simulink model "adc1_sub_start"  (R2018b)
settings: Solver=ode45  StartTime=0.0  StopTime=10.0  RelTol=1e-3  EnableMultiTasking=on
libraries: dsparch4 x2
settings Model: Creator=bbhattac  LastModifiedBy=khung
settings DataIOCC: LimitDataPoints=on  SaveFormat=Array
settings OptimizationCC: ExpressionDepthLimit=2147483647  LifeSpan=inf
settings DebuggingCC: UnderspecifiedInitializationDetection=Classic  MergeDetectMultiDrivingBlocksExec=none  SolverPrmCheckMsg=warning  ParameterPrecisionLossMsg=none  StateNameClashWarn=warning  SFUnexpectedBacktrackingDiag=warning  SFNoUnconditionalDefaultTransitionDiag=warning  SFExecutionAtInitializationDiag=none
settings HardwareCC: ProdBitPerPointer=32  ProdBitPerSizeT=32  ProdBitPerPtrDiffT=32  ProdLargestAtomicFloat=None  ProdIntDivRoundTo=Undefined  ProdEndianess=Unspecified  ProdWordSize=32  ProdHWDeviceType=32-bit Generic
settings ModelReferenceCC: PropagateSignalLabelsOutOfModel=off
settings SFSimCC: SimUseLocalCustomCode=off
settings RTWCC: RTWUseLocalCustomCode=off
settings CodeAppCC: StateflowObjectComments=on
settings GRTTargetCC: TargetLangStandard=C89/C90 (ANSI)  GeneratePreprocessorConditionals=Disable all
settings ConfigComp: CovMetricSettings=dw  CovHtmlReporting=on  CovSaveCumulativeToWorkspaceVar=on  CovSaveSingleToWorkspaceVar=on  CovExternalEMLEnable=off

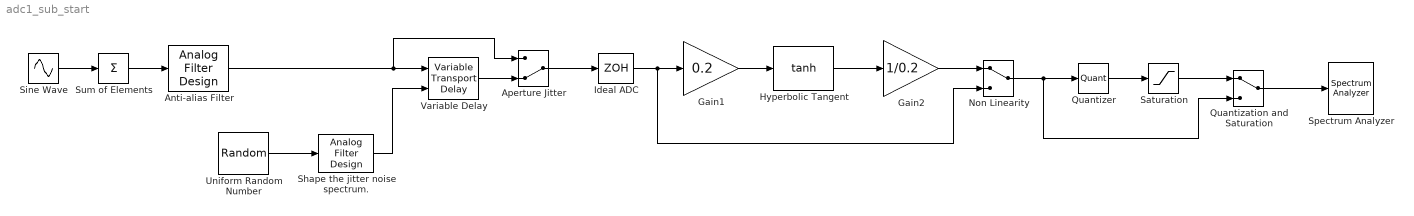
== system adc1_sub_start ==
  Anti-alias Filter : dsparch4/Analog Filter Design  method=Butterworth  filttype=Lowpass  N=8  Wlo=2*pi*50e+06  Whi=80  Rp=2  Rs=40
  Aperture Jitter : ManualSwitch  CurrentSetting=0
  Gain1 : Gain  Gain=0.2  SaturateOnIntegerOverflow=on  OutDataTypeStr=Inherit: Same as input  ParamDataTypeStr=Inherit: Same as input
  Gain2 : Gain  Gain=1/0.2  SaturateOnIntegerOverflow=on  OutDataTypeStr=Inherit: Same as input  ParamDataTypeStr=Inherit: Same as input
  Hyperbolic Tangent : Trigonometry  Operator=tanh
  Ideal ADC : ZeroOrderHold  SampleTime=1/100e6
  Non Linearity : ManualSwitch
  Quantization and Saturation : ManualSwitch
  Quantizer : Quantizer  QuantizationInterval=2^-8
  Saturation : Saturate
  "Shape the jitter noise spectrum. " : dsparch4/Analog Filter Design  method=Butterworth  filttype=Lowpass  N=3  Wlo=2*pi*20e+06  Whi=80  Rp=2  Rs=40
  Sine Wave : Sin  Amplitude=0.25  Frequency=2*pi*[20 22]*1e6  SampleTime=0
  Spectrum Analyzer : SpectrumAnalyzer
  Sum of Elements : Sum  Inputs=+
  Uniform Random Number : UniformRandomNumber  Minimum=0  Maximum=5e-9  Seed=1234  SampleTime=0
  Variable Delay : VariableTransportDelay  MaximumDelay=30e-9  ZeroDelay=on  TransDelayFeedthrough=on
  wires:
  Sine Wave/1 -> Sum of Elements/1
  Sum of Elements/1 -> Anti-alias Filter/1
  Uniform Random Number/1 -> "Shape the jitter noise spectrum. "/1
  "Shape the jitter noise spectrum. "/1 -> Variable Delay/2
  Anti-alias Filter/1 -> Variable Delay/1, Aperture Jitter/1
  Aperture Jitter/1 -> Ideal ADC/1
  Ideal ADC/1 -> Gain1/1, Non Linearity/2
  Variable Delay/1 -> Aperture Jitter/2
  Quantizer/1 -> Saturation/1
  Saturation/1 -> Quantization and Saturation/1
  Non Linearity/1 -> Quantization and Saturation/2, Quantizer/1
  Quantization and Saturation/1 -> Spectrum Analyzer/1
  Gain2/1 -> Non Linearity/1
  Hyperbolic Tangent/1 -> Gain2/1
  Gain1/1 -> Hyperbolic Tangent/1
